simulink model "ME416_Autonomy_Model_Rollback2"  (R2025b)
settings: Solver=FixedStepAuto  StartTime=0.0  StopTime=240  RelTol=1e-3  EnableMultiTasking=on
PreLoadFcn:
  | driveparam
values from neighbouring files (symbols this model uses):
  alpha_w = 0.7    [driveparam.m]
  beta = Ts / (Ts + tau)    (= 0.166666666667)    [driveparam.m]
  enable_cmd = 1    [driveparam.m]
  estop_cmd = 0    [driveparam.m]
  K_lqr_w = dlqr(Ad_w, Bd_w, Qw, Rw)    [driveparam.m]
  L = 0.15    [driveparam.m]
  N = 4400    [driveparam.m]
  Nbar_lqr_w = (1 - Ad_w)/Bd_w + K_lqr_w    [driveparam.m]
  r = 0.03    [driveparam.m]
  Ts = 0.01    [driveparam.m]
  v_ref_cmd = 0    [driveparam.m]
  w_ref_cmd = 0.1    [driveparam.m]
undefined symbols (not defined in the file or in its folder): DiscIntNeverNeededParam, dspblkCoreblockFVToolHelper, gcbh
libraries: raspberrypiBasiclib x22, simulink x21, raspberrypiCommlib x19, slpidlib x2
(part 3 of 3)

== matlab function ME416_Autonomy_Model_Rollback2/HardwareIO/IMU_System/MATLAB Function1 ==
  data: ax_parsed input; ax_kf output; ay_parsed input; az_parsed input; ay_kf output; az_kf output; pitch_kf output; roll_kf output
function [ax_kf, ay_kf, az_kf, pitch_kf, roll_kf] = mma8451_kalman_filter(ax_parsed, ay_parsed, az_parsed)
%#codegen
% Simple 1D Kalman smoothing filter for 3-axis accelerometer
%
% Inputs:
%   ax, ay, az   -> accelerometer in g
%
% Outputs:
%   ax_kf, ay_kf, az_kf     -> filtered accel
%   pitch_kf, roll_kf       -> filtered angles from accel

% Persistent states for each filtered signal
persistent x_ax_parsed p_ax_parsed
persistent x_ay_parsed p_ay_parsed
persistent x_az_parsed p_az_parsed
persistent x_pitch p_pitch
persistent x_roll p_roll

% Tunable Kalman parameters
% Lower q = smoother/slower
% Lower r = trusts measurement more
q_acc = 0.001; r_acc = 0.2;
q_ang = 0.001; r_ang = 0.2;

% Compute raw roll/pitch from accelerometer
roll_meas  = atan2(ay_parsed, az_parsed);
pitch_meas = atan2(-ax_parsed, sqrt(ay_parsed^2 + az_parsed^2));

% Initialize on first run
if isempty(x_ax_parsed)
    x_ax_parsed = ax_parsed;      p_ax_parsed = 1.0;
    x_ay_parsed = ay_parsed;      p_ay_parsed = 1.0;
    x_az_parsed = az_parsed;      p_az_parsed = 1.0;
    x_roll  = roll_meas;          p_roll  = 1.0;
    x_pitch = pitch_meas;         p_pitch = 1.0;
end

% Filter accel channels
[x_ax_parsed, p_ax_parsed] = kalman_update(x_ax_parsed, p_ax_parsed, ax_parsed, q_acc, r_acc);
[x_ay_parsed, p_ay_parsed] = kalman_update(x_ay_parsed, p_ay_parsed, ay_parsed, q_acc, r_acc);
[x_az_parsed, p_az_parsed] = kalman_update(x_az_parsed, p_az_parsed, az_parsed, q_acc, r_acc);

% Filter roll/pitch angles
[x_roll, p_roll]   = kalman_update(x_roll, p_roll, roll_meas, q_ang, r_ang);
[x_pitch, p_pitch] = kalman_update(x_pitch, p_pitch, pitch_meas, q_ang, r_ang);

% Outputs
ax_kf = x_ax_parsed;
ay_kf = x_ay_parsed;
az_kf = x_az_parsed;
roll_kf  = x_roll;
pitch_kf = x_pitch;
end

function [x, p] = kalman_update(x, p, z, q, r)
% 1D Kalman filter update
% Prediction
p = p + q;
% Correction
k = p / (p + r);
x = x + k * (z - x);
p = (1 - k) * p;
end

== matlab function ME416_Autonomy_Model_Rollback2/HardwareIO/IMU_System/MPU6050_Parse_Function ==
  data: bytes input; ax output; ay output; az output; gx output; gy output; gz output
function [ax, ay, az, gx, gy, gz] = parse_mpu6050(bytes)
%#codegen
% bytes: 14x1 uint8 from MPU6050 starting at 0x3B

ax_raw = combineSigned(bytes(1),  bytes(2));
ay_raw = combineSigned(bytes(3),  bytes(4));
az_raw = combineSigned(bytes(5),  bytes(6));

gx_raw = combineSigned(bytes(9),  bytes(10));
gy_raw = combineSigned(bytes(11), bytes(12));
gz_raw = combineSigned(bytes(13), bytes(14));

% Scale assuming accel +/-2g, gyro +/-250 deg/s
ax = double(ax_raw) / 16384.0;
ay = double(ay_raw) / 16384.0;
az = double(az_raw) / 16384.0;

gx = double(gx_raw) / 131.0 * (pi / 180.0);
gy = double(gy_raw) / 131.0 * (pi / 180.0);
gz = double(gz_raw) / 131.0 * (pi / 180.0);

end

function x = combineSigned(hi, lo)
% hi, lo are uint8
u = bitor(bitshift(uint16(hi), 8), uint16(lo));

if u >= 32768
    x = int16(int32(u) - 65536);
else
    x = int16(u);
end
end

== matlab function ME416_Autonomy_Model_Rollback2/HardwareIO/IMU_System/IMU1_Kalman_Filter ==
  data: ax_parsed input; ax_kf output; ay_parsed input; az_parsed input; gx_parsed input; ay_kf output; az_kf output; pitch_kf output; roll_kf output; yaw_rate_kf output; gy_parsed input; gz_parsed input
function [ax_kf, ay_kf, az_kf, pitch_kf, roll_kf, yaw_rate_kf] = imu_kalman_filter(ax_parsed, ay_parsed, az_parsed, gx_parsed, gy_parsed, gz_parsed)
%#codegen
% Simple 1D Kalman smoothing filter for IMU signals
%
% Inputs:
%   ax, ay, az   -> accelerometer in g
%   gx, gy, gz   -> gyro in rad/sa
%
% Outputs:
%   ax_f, ay_f, az_f     -> filtered accel
%   pitch_f, roll_f      -> filtered angles from accel
%   yaw_rate_f           -> filtered yaw rate from gyro z

% Persistent states for each filtered signal
persistent x_ax_parsed p_ax_parsed
persistent x_ay_parsed p_ay_parsed
persistent x_az_parsed p_az_parsed
persistent x_pitch p_pitch
persistent x_roll p_roll
persistent x_yaw p_yaw

% Tunable Kalman parameters
% Lower q = smoother/slower
% Lower r = trusts measurement more
q_acc = 0.001; r_acc = 0.2;
q_ang = 0.001; r_ang = 0.2;
q_yaw = 0.001; r_yaw = 0.3;

% Compute raw roll/pitch from accelerometer
roll_meas  = atan2(ay_parsed, az_parsed);
pitch_meas = atan2(-ax_parsed, sqrt(ay_parsed^2 + az_parsed^2));

% Initialize on first run
if isempty(x_ax_parsed)
    x_ax_parsed = ax_parsed;      p_ax_parsed = 1.0;
    x_ay_parsed = ay_parsed;      p_ay_parsed = 1.0;
    x_az_parsed = az_parsed;      p_az_parsed = 1.0;

    x_roll  = roll_meas;    p_roll  = 1.0;
    x_pitch = pitch_meas;   p_pitch = 1.0;

    x_yaw = gz_parsed;      p_yaw = 1.0;
end

% Filter accel channels
[x_ax_parsed, p_ax_parsed] = kalman_update(x_ax_parsed, p_ax_parsed, ax_parsed, q_acc, r_acc);
[x_ay_parsed, p_ay_parsed] = kalman_update(x_ay_parsed, p_ay_parsed, ay_parsed, q_acc, r_acc);
[x_az_parsed, p_az_parsed] = kalman_update(x_az_parsed, p_az_parsed, az_parsed, q_acc, r_acc);

% Filter roll/pitch angles
[x_roll, p_roll]   = kalman_update(x_roll, p_roll, roll_meas, q_ang, r_ang);
[x_pitch, p_pitch] = kalman_update(x_pitch, p_pitch, pitch_meas, q_ang, r_ang);

% Filter yaw rate (gyro z)
[x_yaw, p_yaw] = kalman_update(x_yaw, p_yaw, gz_parsed, q_yaw, r_yaw);

% Outputs
ax_kf = x_ax_parsed;
ay_kf = x_ay_parsed;
az_kf = x_az_parsed;

roll_kf     = x_roll;
pitch_kf    = x_pitch;
yaw_rate_kf = x_yaw;

end

function [x, p] = kalman_update(x, p, z, q, r)
% 1D Kalman filter update

% Prediction
p = p + q;

% Correction
k = p / (p + r);
x = x + k * (z - x);
p = (1 - k) * p;

end

== matlab function ME416_Autonomy_Model_Rollback2/HardwareIO/IMU_System/IMU2_Kalman_Filter ==
  data: ax_parsed input; ax_kf output; ay_parsed input; az_parsed input; gx_parsed input; ay_kf output; az_kf output; pitch_kf output; roll_kf output; yaw_rate_kf output; gy_parsed input; gz_parsed input
function [ax_kf, ay_kf, az_kf, pitch_kf, roll_kf, yaw_rate_kf] = imu_kalman_filter(ax_parsed, ay_parsed, az_parsed, gx_parsed, gy_parsed, gz_parsed)
%#codegen
% Simple 1D Kalman smoothing filter for IMU signals
%
% Inputs:
%   ax, ay, az   -> accelerometer in g
%   gx, gy, gz   -> gyro in rad/sa
%
% Outputs:
%   ax_f, ay_f, az_f     -> filtered accel
%   pitch_f, roll_f      -> filtered angles from accel
%   yaw_rate_f           -> filtered yaw rate from gyro z

% Persistent states for each filtered signal
persistent x_ax_parsed p_ax_parsed
persistent x_ay_parsed p_ay_parsed
persistent x_az_parsed p_az_parsed
persistent x_pitch p_pitch
persistent x_roll p_roll
persistent x_yaw p_yaw

% Tunable Kalman parameters
% Lower q = smoother/slower
% Lower r = trusts measurement more
q_acc = 0.001; r_acc = 0.2;
q_ang = 0.001; r_ang = 0.2;
q_yaw = 0.001; r_yaw = 0.3;

% Compute raw roll/pitch from accelerometer
roll_meas  = atan2(ay_parsed, az_parsed);
pitch_meas = atan2(-ax_parsed, sqrt(ay_parsed^2 + az_parsed^2));

% Initialize on first run
if isempty(x_ax_parsed)
    x_ax_parsed = ax_parsed;      p_ax_parsed = 1.0;
    x_ay_parsed = ay_parsed;      p_ay_parsed = 1.0;
    x_az_parsed = az_parsed;      p_az_parsed = 1.0;

    x_roll  = roll_meas;    p_roll  = 1.0;
    x_pitch = pitch_meas;   p_pitch = 1.0;

    x_yaw = gz_parsed;      p_yaw = 1.0;
end

% Filter accel channels
[x_ax_parsed, p_ax_parsed] = kalman_update(x_ax_parsed, p_ax_parsed, ax_parsed, q_acc, r_acc);
[x_ay_parsed, p_ay_parsed] = kalman_update(x_ay_parsed, p_ay_parsed, ay_parsed, q_acc, r_acc);
[x_az_parsed, p_az_parsed] = kalman_update(x_az_parsed, p_az_parsed, az_parsed, q_acc, r_acc);

% Filter roll/pitch angles
[x_roll, p_roll]   = kalman_update(x_roll, p_roll, roll_meas, q_ang, r_ang);
[x_pitch, p_pitch] = kalman_update(x_pitch, p_pitch, pitch_meas, q_ang, r_ang);

% Filter yaw rate (gyro z)
[x_yaw, p_yaw] = kalman_update(x_yaw, p_yaw, gz_parsed, q_yaw, r_yaw);

% Outputs
ax_kf = x_ax_parsed;
ay_kf = x_ay_parsed;
az_kf = x_az_parsed;

roll_kf     = x_roll;
pitch_kf    = x_pitch;
yaw_rate_kf = x_yaw;

end

function [x, p] = kalman_update(x, p, z, q, r)
% 1D Kalman filter update

% Prediction
p = p + q;

% Correction
k = p / (p + r);
x = x + k * (z - x);
p = (1 - k) * p;

end

== matlab function ME416_Autonomy_Model_Rollback2/HardwareIO/IMU_System/MPU6050_Parse_Function1 ==
  data: bytes input; ax output; ay output; az output; gx output; gy output; gz output
function [ax, ay, az, gx, gy, gz] = parse_mpu6050(bytes)
%#codegen
% bytes: 14x1 uint8 from MPU6050 starting at 0x3B

ax_raw = combineSigned(bytes(1),  bytes(2));
ay_raw = combineSigned(bytes(3),  bytes(4));
az_raw = combineSigned(bytes(5),  bytes(6));

gx_raw = combineSigned(bytes(9),  bytes(10));
gy_raw = combineSigned(bytes(11), bytes(12));
gz_raw = combineSigned(bytes(13), bytes(14));

% Scale assuming accel +/-2g, gyro +/-250 deg/s
ax = double(ax_raw) / 16384.0;
ay = double(ay_raw) / 16384.0;
az = double(az_raw) / 16384.0;

gx = double(gx_raw) / 131.0 * (pi / 180.0);
gy = double(gy_raw) / 131.0 * (pi / 180.0);
gz = double(gz_raw) / 131.0 * (pi / 180.0);

end

function x = combineSigned(hi, lo)
% hi, lo are uint8
u = bitor(bitshift(uint16(hi), 8), uint16(lo));

if u >= 32768
    x = int16(int32(u) - 65536);
else
    x = int16(u);
end
end
